simulink model "simulinku"  (R2023b)
settings: Solver=FixedStepAuto  StartTime=0.0  StopTime=100  FixedStep=0.1  RelTol=1e-3
values from neighbouring files (symbols this model uses):
  Hc_d = c2d(Hpi,0.1,'zoh')    [lab2.m]
  Hd_d = c2d(Hpd,0.1,'zoh')    [lab2.m]
  Hp = tf(num,den,'IOdelay',1)    [lab2.m]
  Hp_d = c2d(Hp,0.1,'zoh')    [lab2.m]
  Hpd = kd * (tf([Td 1],[Td*beta 1]))    [lab2.m]
  Hpi = kpi * (1 + tf([1],[Ti 0]))    [lab2.m]
settings Model: Creator=Cristi  LastModifiedBy=Cristi

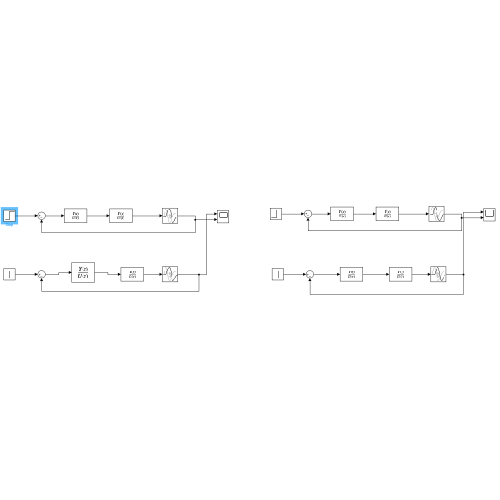
[thumbnail: Simulink's stored preview of the top-level diagram]
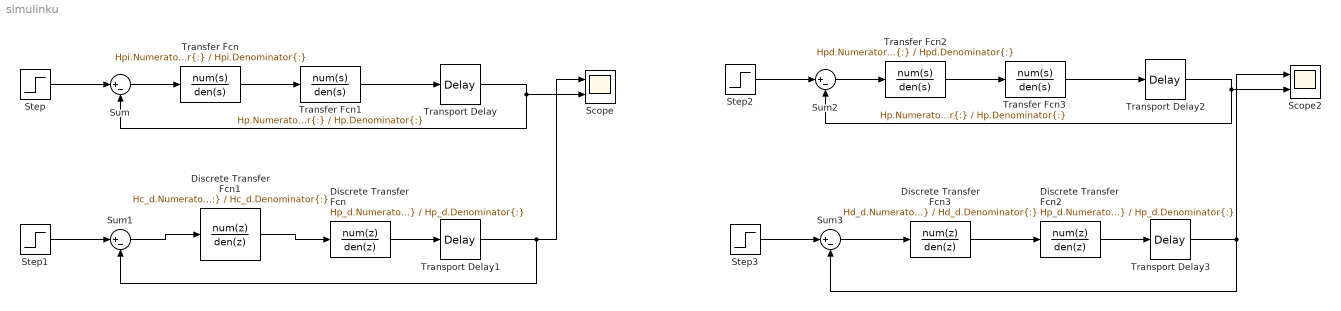
== system simulinku ==
  Discrete Transfer Fcn : DiscreteTransferFcn  Numerator=Hp_d.Numerator{:}  Denominator=Hp_d.Denominator{:}
  Discrete Transfer Fcn1 : DiscreteTransferFcn  Numerator=Hc_d.Numerator{:}  Denominator=Hc_d.Denominator{:}
  Discrete Transfer Fcn2 : DiscreteTransferFcn  Numerator=Hp_d.Numerator{:}  Denominator=Hp_d.Denominator{:}
  Discrete Transfer Fcn3 : DiscreteTransferFcn  Numerator=Hd_d.Numerator{:}  Denominator=Hd_d.Denominator{:}
  Scope : Scope  NumInputPorts=2
  Scope2 : Scope  NumInputPorts=2
  Step{,1..3} (4 alike) : Step  Time=50  Before=15  After=17  SampleTime=0
  Sum{,1..3} (4 alike) : Sum  Inputs=|+-
  Transfer Fcn : TransferFcn  Numerator=Hpi.Numerator{:}  Denominator=Hpi.Denominator{:}
  Transfer Fcn1 : TransferFcn  Numerator=Hp.Numerator{:}  Denominator=Hp.Denominator{:}
  Transfer Fcn2 : TransferFcn  Numerator=Hpd.Numerator{:}  Denominator=Hpd.Denominator{:}
  Transfer Fcn3 : TransferFcn  Numerator=Hp.Numerator{:}  Denominator=Hp.Denominator{:}
  Transport Delay{,1..3} (4 alike) : TransportDelay
  wires:
  Transport Delay/1 -> Sum/2, Scope/2
  Sum/1 -> Transfer Fcn/1
  Transfer Fcn/1 -> Transfer Fcn1/1
  Transfer Fcn1/1 -> Transport Delay/1
  Transport Delay1/1 -> Scope/1, Sum1/2
  Step1/1 -> Sum1/1
  Sum1/1 -> Discrete Transfer Fcn1/1
  Discrete Transfer Fcn1/1 -> Discrete Transfer Fcn/1
  Discrete Transfer Fcn/1 -> Transport Delay1/1
  Step/1 -> Sum/1
  Transfer Fcn2/1 -> Transfer Fcn3/1
  Sum2/1 -> Transfer Fcn2/1
  Transport Delay2/1 -> Sum2/2, Scope2/2
  Step2/1 -> Sum2/1
  Transfer Fcn3/1 -> Transport Delay2/1
  Discrete Transfer Fcn2/1 -> Transport Delay3/1
  Step3/1 -> Sum3/1
  Discrete Transfer Fcn3/1 -> Discrete Transfer Fcn2/1
  Transport Delay3/1 -> Sum3/2, Scope2/1
  Sum3/1 -> Discrete Transfer Fcn3/1
